simulink library "lib_electric_machine"  (Simulink 4.1.1)
undefined symbols (not defined in the file or in its folder): amb_tmp, cyc_mph, ess_module_num, ess_voc, fd_ratio, gb_num_init, gb_ratio, gc_cp, gc_inertia, gc_inpwr_map, gc_map_spd, gc_map_trq, gc_mass, gc_max_crrnt, gc_max_trq, gc_outpwr_map, gc_overtrq_factor, gc_sarea, gc_spd_scale, gc_th_calc, gc_trq_scale, gc_tstat, mc_cp, mc_eff_scale, mc_inertia, mc_init_tmp, mc_inpwr_map, mc_map_spd, mc_map_trq, mc_mass, mc_max_gen_trq, mc_max_trq, mc_overtrq_factor, mc_sarea, mc_spd_scale, mc_th_calc, mc_trq_scale, mc_tstat, tc_mc_to_fc_ratio, veh_mass, wh_radius
libraries: lib_electric_machine x4
(part 1 of 2)
settings Model: LastModifiedBy=ssprik
settings Model: ModifiedComment=|
  | abrooker -- Wed Aug 13 10:56:21 2003 -- Version 1.20
  | changed mc_eff_scale implementation into model
settings Model: ModifiedHistory=|
  | abrooker -- Tue Feb 04 10:35:40 2003 -- Version 1.19
  | added pwr goto for Altia
  | 
  | mokeefe -- Thu Apr 18 08:27:13 2002 -- Version 1.18
  | saving the model:
  | o "without the model browser open"
  | o with only top-level screen visible
  | o with "fit to view" enabled
  | o with "status bar" off and "toolbar" off
  | o with "prompt to update model history with each save" on

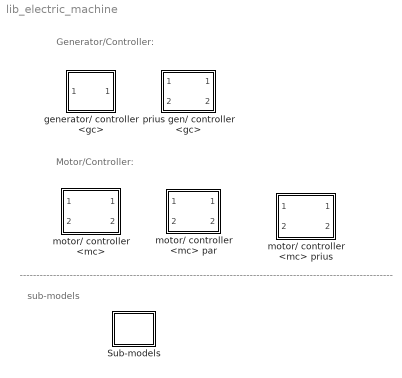
== system lib_electric_machine ==
  note: Generator/Controller:
  note: Motor/Controller:
  note: ----------------------------------------------------------------------------------------------------------------
  note: sub-models
  Sub-models : Subsystem
      settings: RTWFcnNameOpts=Auto  RTWFileNameOpts=Auto
  generator/ controller <gc> : Subsystem
      settings: RTWFcnNameOpts=Auto  RTWFileNameOpts=Auto
      mask Display: image(imread('bdi_mc.jpg'))
  motor/ controller <mc> : Subsystem
      settings: RTWFcnNameOpts=Auto  RTWFileNameOpts=Auto
      mask Display: image(imread('bdi_mc.jpg'))
  motor/ controller <mc> par : Subsystem
      settings: RTWFcnNameOpts=Auto  RTWFileNameOpts=Auto
      mask Display: image(imread('bdi_mc.jpg'))
  motor/ controller <mc> prius : Subsystem
      settings: RTWFcnNameOpts=Auto  RTWFileNameOpts=Auto
      mask Display: image(imread('bdi_mc.jpg'))
  prius gen/ controller <gc> : Subsystem
      settings: RTWFcnNameOpts=Auto  RTWFileNameOpts=Auto
      mask Display: image(imread('bdi_mc.jpg'))

== system lib_electric_machine/Sub-models ==
  motor inertia as a function of total vehicle inertia (generous approximation) : Subsystem  Orientation=up
      settings: RTWFcnNameOpts=Auto  RTWFileNameOpts=Auto
  veh mass calc : Subsystem
      settings: RTWFcnNameOpts=Auto  RTWFileNameOpts=Auto

== system lib_electric_machine/generator/ controller <gc> ==
  "torque and speed supplied to rotor (Nm), (rad/s)" : Inport  Port=1  LatchInput=off
  >=0 : Saturate  UpperLimit=inf  LowerLimit=0  LinearizeAsGain=on
  Block NOTES : Subsystem
      settings: RTWFcnNameOpts=Auto  RTWFileNameOpts=Auto
      mask Display: disp('Block\nNOTES')
  Demux : Demux  Outputs=2  BusSelectionMode=off
  Memory : Memory  X0=ess_module_num*mean(ess_voc(1,:))  InheritSampleTime=off
      settings: RTWStateStorageClass=Auto
  Sum : Sum  Inputs=+-  SaturateOnIntegerOverflow=on
  To Workspace9 : ToWorkspace  VariableName=gc_pwr_out_a  SampleTime=-1  SaveFormat=Array
      settings: Orientation=down
  effect of inertia (Nm) : Subsystem
      settings: RTWFcnNameOpts=Auto  RTWFileNameOpts=Auto
  enforce torque limit : Subsystem
      settings: RTWFcnNameOpts=Auto  RTWFileNameOpts=Auto
  enforce max speed : Saturate  UpperLimit=max(gc_map_spd)*gc_spd_scale  LowerLimit=0  LinearizeAsGain=on
  generator output power map (W) : Lookup2D  RowIndex=gc_map_spd*gc_spd_scale  ColumnIndex=gc_map_trq*gc_trq_scale  OutputValues=gc_outpwr_map*gc_spd_scale*gc_trq_scale
  help : Subsystem
      settings: OpenFcn=web(['file:\\\' which('generator_controller.htm')]);  RTWFcnNameOpts=Auto  RTWFileNameOpts=Auto
      mask Display: image(imread('doc_man.jpg'))
  limit request: controller current limit : Subsystem
      settings: RTWFcnNameOpts=Auto  RTWFileNameOpts=Auto
  generator output power (W) : Outport  Port=1  InitialOutput=0
  tag scope: gc_pwr_out_a=global, gc_spd_in_a=global, gc_trq_in_a=global
  wires:
  >=0/1 -> generator output power (W)/1, To Workspace9/1, [gc_pwr_out_a]
  limit request: controller current limit/1(out_1) -> >=0/1
  Demux/1 -> Sum/1, [gc_trq_in_a]
  [bus_voltage] -> Memory/1
  enforce max speed/1 -> generator output power map (W)/1, enforce torque limit/2(limited generator speed (rad/s))
  generator output power map (W)/1 -> limit request: controller current limit/1(computed output power (W))
  Sum/1 -> enforce torque limit/1(req'd generator input torque (Nm))
  enforce torque limit/1(limited generator input torque (Nm)) -> generator output power map (W)/2
  effect of inertia (Nm)/1(out_1) -> Sum/2
  Memory/1 -> limit request: controller current limit/2(bus voltage (V))
  "torque and speed supplied to rotor (Nm), (rad/s)"/1 -> Demux/1
  Demux/2 -> effect of inertia (Nm)/1(in_1), enforce max speed/1, [gc_spd_in_a]

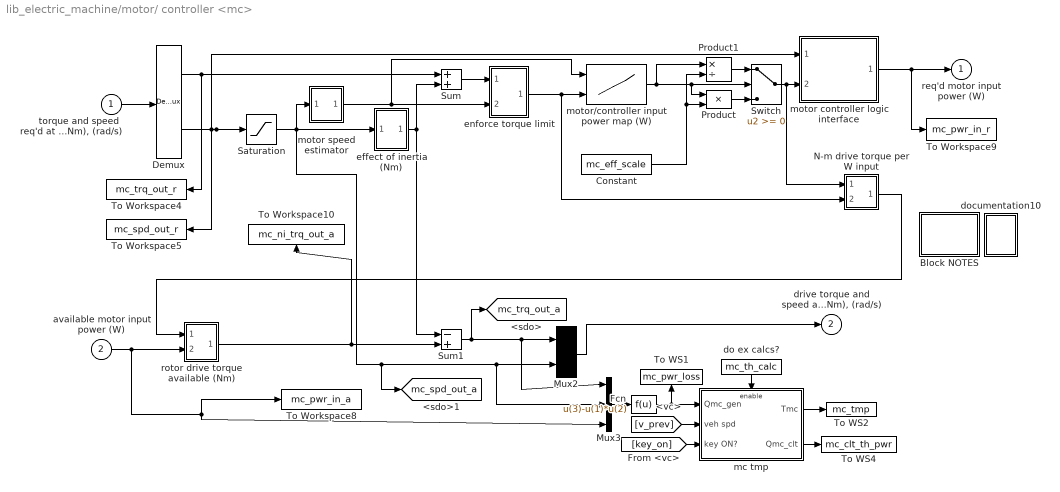
== system lib_electric_machine/motor/ controller <mc> ==
  "torque and speed  req'd at rotor (Nm), (rad/s)" : Inport  Port=1  LatchInput=off
  available motor input power (W) : Inport  Port=2  LatchInput=off
  Block NOTES : Subsystem
      settings: RTWFcnNameOpts=Auto  RTWFileNameOpts=Auto
      mask Display: disp('Block\nNOTES')
  Constant : Constant  Value=mc_eff_scale
  Demux : Demux  Outputs=2  BusSelectionMode=off
  Fcn : Fcn  Expr=u(3)-u(1)*u(2)
  Mux2 : Mux  Inputs=2
      settings: DisplayOption=none
  Mux3 : Mux  Inputs=3
      settings: DisplayOption=none
  N-m drive torque per W input : Subsystem
      settings: RTWFcnNameOpts=Auto  RTWFileNameOpts=Auto
  Product : Product  Inputs=2  Multiplication=Element-wise(.*)  SaturateOnIntegerOverflow=on
  Product1 : Product  Inputs=*/  Multiplication=Element-wise(.*)  SaturateOnIntegerOverflow=on
  Saturation : Saturate  UpperLimit=max(mc_map_spd)*mc_spd_scale  LowerLimit=0  LinearizeAsGain=on
  Sum : Sum  Inputs=++  SaturateOnIntegerOverflow=on
  Sum1 : Sum  Inputs=-+  SaturateOnIntegerOverflow=on
  Switch : Switch  Threshold=0
  To WS1 : ToWorkspace  VariableName=mc_pwr_loss  SampleTime=0  SaveFormat=Array
      settings: Orientation=up  MaxDataPoints=50000
  To WS2 : ToWorkspace  VariableName=mc_tmp  SampleTime=0  SaveFormat=Array
      settings: MaxDataPoints=50000
  To WS4 : ToWorkspace  VariableName=mc_clt_th_pwr  SampleTime=0  SaveFormat=Array
      settings: MaxDataPoints=50000
  To Workspace10 : ToWorkspace  VariableName=mc_ni_trq_out_a  SampleTime=-1  SaveFormat=Array
      settings: Orientation=up
  To Workspace4 : ToWorkspace  VariableName=mc_trq_out_r  SampleTime=-1  SaveFormat=Array
  To Workspace5 : ToWorkspace  VariableName=mc_spd_out_r  SampleTime=-1  SaveFormat=Array
  To Workspace8 : ToWorkspace  VariableName=mc_pwr_in_a  SampleTime=-1  SaveFormat=Array
  To Workspace9 : ToWorkspace  VariableName=mc_pwr_in_r  SampleTime=-1  SaveFormat=Array
  do ex calcs? : Constant  Orientation=down  Value=mc_th_calc
  documentation10 : Subsystem
      settings: OpenFcn=web(['file:\\\' which('motor_controller.htm')]);  RTWFcnNameOpts=Auto  RTWFileNameOpts=Auto
      mask Display: image(imread('doc_man.jpg'))
  effect of inertia (Nm) : Subsystem
      settings: RTWFcnNameOpts=Auto  RTWFileNameOpts=Auto
  enforce torque limit : Subsystem
      settings: RTWFcnNameOpts=Auto  RTWFileNameOpts=Auto
  mc tmp : Subsystem  TreatAsAtomicUnit=on
      settings: RTWFcnNameOpts=Auto  RTWFileNameOpts=Auto
  motor controller logic interface : Subsystem
      settings: RTWFcnNameOpts=Auto  RTWFileNameOpts=Auto
  motor speed estimator : Subsystem
      settings: RTWFcnNameOpts=Auto  RTWFileNameOpts=Auto
  motor/controller input power map (W) : Lookup2D  RowIndex=mc_map_spd*mc_spd_scale  ColumnIndex=mc_map_trq*mc_trq_scale  OutputValues=mc_inpwr_map*mc_spd_scale*mc_trq_scale
  rotor drive torque available (Nm) : Subsystem
      settings: RTWFcnNameOpts=Auto  RTWFileNameOpts=Auto
  req'd motor input power (W) : Outport  Port=1  InitialOutput=0
  "drive torque and speed avail. at rotor (Nm), (rad/s)" : Outport  Port=2  InitialOutput=0
  tag scope: mc_spd_out_a=global, mc_trq_out_a=global
  wires:
  "torque and speed  req'd at rotor (Nm), (rad/s)"/1 -> Demux/1
  Demux/1 -> To Workspace4/1, Sum/1
  available motor input power (W)/1 -> rotor drive torque available (Nm)/2(available input power (W)), To Workspace8/1, Mux3/3
  Demux/2 -> motor controller logic interface/1(w_mc_out_r), To Workspace5/1, Saturation/1
  [key_on] -> mc tmp/3(key ON?)
  [v_prev] -> mc tmp/2(veh spd)
  mc tmp/2(Qmc_clt) -> To WS4/1
  mc tmp/1(Tmc) -> To WS2/1
  do ex calcs?/1 -> mc tmp/Enable
  Fcn/1 -> mc tmp/1(Qmc_gen), To WS1/1
  Mux3/1 -> Fcn/1
  Mux2/1 -> "drive torque and speed avail. at rotor (Nm), (rad/s)"/1
  motor controller logic interface/1(P_mc_in_r) -> req'd motor input power (W)/1, To Workspace9/1
  enforce torque limit/1(limited motor torque (Nm)) -> N-m drive torque per W input/2(req'd rotor drive torque (Nm)), motor/controller input power map (W)/2
  effect of inertia (Nm)/1(out_1) -> Sum1/1, Sum/2
  Sum/1 -> enforce torque limit/1(req'd motor torque (Nm))
  Sum1/1 -> [mc_trq_out_a], Mux2/1, Mux3/1
  Saturation/1 -> motor speed estimator/1(mc_spd_out_a), effect of inertia (Nm)/1(mc_spd_out_a), [mc_spd_out_a], Mux2/2, Mux3/2
  motor speed estimator/1(Out1) -> enforce torque limit/2(limited motor speed (rad/s)), motor/controller input power map (W)/1
  N-m drive torque per W input/1(Nm per W) -> rotor drive torque available (Nm)/1(torque per unit input power (N-m/W))
  rotor drive torque available (Nm)/1(rotor drive torque available) -> To Workspace10/1, Sum1/2
  Switch/1 -> motor controller logic interface/2(P_mc_in_1lim), N-m drive torque per W input/1(req'd input power (W))
  Product1/1 -> Switch/1
  motor/controller input power map (W)/1 -> Product1/1, Switch/2, Product/1
  Constant/1 -> Product1/2, Product/2
  Product/1 -> Switch/3

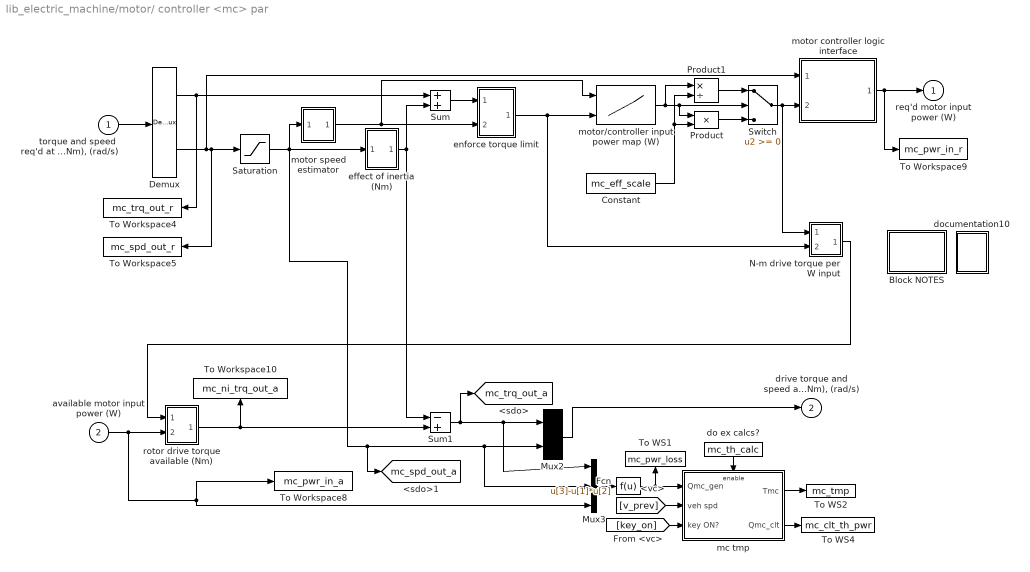
== system lib_electric_machine/motor/ controller <mc> par ==
  "torque and speed  req'd at rotor (Nm), (rad/s)" : Inport  Port=1  LatchInput=off
  available motor input power (W) : Inport  Port=2  LatchInput=off
  Block NOTES : Subsystem
      settings: RTWFcnNameOpts=Auto  RTWFileNameOpts=Auto
      mask Display: disp('Block\nNOTES')
  Constant : Constant  Value=mc_eff_scale
  Demux : Demux  Outputs=2  BusSelectionMode=off
  Fcn : Fcn  Expr=u[3]-u[1]*u[2]
  Mux2 : Mux  Inputs=2
      settings: DisplayOption=none
  Mux3 : Mux  Inputs=3
      settings: DisplayOption=none
  N-m drive torque per W input : Subsystem
      settings: RTWFcnNameOpts=Auto  RTWFileNameOpts=Auto
  Product : Product  Inputs=2  Multiplication=Element-wise(.*)  SaturateOnIntegerOverflow=on
  Product1 : Product  Inputs=*/  Multiplication=Element-wise(.*)  SaturateOnIntegerOverflow=on
  Saturation : Saturate  UpperLimit=max(mc_map_spd)*mc_spd_scale  LowerLimit=0  LinearizeAsGain=on
  Sum : Sum  Inputs=++  SaturateOnIntegerOverflow=on
  Sum1 : Sum  Inputs=-+  SaturateOnIntegerOverflow=on
  Switch : Switch  Threshold=0
  To WS1 : ToWorkspace  VariableName=mc_pwr_loss  SampleTime=0  SaveFormat=Array
      settings: Orientation=up  MaxDataPoints=50000
  To WS2 : ToWorkspace  VariableName=mc_tmp  SampleTime=0  SaveFormat=Array
      settings: MaxDataPoints=50000
  To WS4 : ToWorkspace  VariableName=mc_clt_th_pwr  SampleTime=0  SaveFormat=Array
      settings: MaxDataPoints=50000
  To Workspace10 : ToWorkspace  VariableName=mc_ni_trq_out_a  SampleTime=-1  SaveFormat=Array
      settings: Orientation=up
  To Workspace4 : ToWorkspace  VariableName=mc_trq_out_r  SampleTime=-1  SaveFormat=Array
  To Workspace5 : ToWorkspace  VariableName=mc_spd_out_r  SampleTime=-1  SaveFormat=Array
  To Workspace8 : ToWorkspace  VariableName=mc_pwr_in_a  SampleTime=-1  SaveFormat=Array
  To Workspace9 : ToWorkspace  VariableName=mc_pwr_in_r  SampleTime=-1  SaveFormat=Array
  do ex calcs? : Constant  Orientation=down  Value=mc_th_calc
  documentation10 : Subsystem
      settings: OpenFcn=web(['file:\\\' which('motor_controller.htm')]);  RTWFcnNameOpts=Auto  RTWFileNameOpts=Auto
      mask Display: image(imread('doc_man.jpg'))
  effect of inertia (Nm) : Subsystem
      settings: RTWFcnNameOpts=Auto  RTWFileNameOpts=Auto
  enforce torque limit : Subsystem
      settings: RTWFcnNameOpts=Auto  RTWFileNameOpts=Auto
  mc tmp : Subsystem  TreatAsAtomicUnit=on
      settings: RTWFcnNameOpts=Auto  RTWFileNameOpts=Auto
  motor controller logic interface : Subsystem
      settings: RTWFcnNameOpts=Auto  RTWFileNameOpts=Auto
  motor speed estimator : Subsystem
      settings: RTWFcnNameOpts=Auto  RTWFileNameOpts=Auto
  motor/controller input power map (W) : Lookup2D  RowIndex=mc_map_spd*mc_spd_scale  ColumnIndex=mc_map_trq*mc_trq_scale  OutputValues=mc_inpwr_map*mc_spd_scale*mc_trq_scale
  rotor drive torque available (Nm) : Subsystem
      settings: RTWFcnNameOpts=Auto  RTWFileNameOpts=Auto
  req'd motor input power (W) : Outport  Port=1  InitialOutput=0
  "drive torque and speed avail. at rotor (Nm), (rad/s)" : Outport  Port=2  InitialOutput=0
  tag scope: mc_spd_out_a=global, mc_trq_out_a=global
  wires:
  rotor drive torque available (Nm)/1(rotor drive torque available) -> To Workspace10/1, Sum1/2
  "torque and speed  req'd at rotor (Nm), (rad/s)"/1 -> Demux/1
  Demux/1 -> To Workspace4/1, Sum/1
  available motor input power (W)/1 -> rotor drive torque available (Nm)/2(available input power (W)), To Workspace8/1, Mux3/3
  Demux/2 -> motor controller logic interface/1(w_mc_out_r), To Workspace5/1, Saturation/1
  [key_on] -> mc tmp/3(key ON?)
  [v_prev] -> mc tmp/2(veh spd)
  mc tmp/2(Qmc_clt) -> To WS4/1
  mc tmp/1(Tmc) -> To WS2/1
  do ex calcs?/1 -> mc tmp/Enable
  Fcn/1 -> mc tmp/1(Qmc_gen), To WS1/1
  Mux3/1 -> Fcn/1
  Mux2/1 -> "drive torque and speed avail. at rotor (Nm), (rad/s)"/1
  motor controller logic interface/1(P_mc_in_r) -> req'd motor input power (W)/1, To Workspace9/1
  enforce torque limit/1(limited motor torque (Nm)) -> motor/controller input power map (W)/2, N-m drive torque per W input/2(req'd rotor drive torque (Nm))
  effect of inertia (Nm)/1(out_1) -> Sum1/1, Sum/2
  Sum/1 -> enforce torque limit/1(req'd motor torque (Nm))
  N-m drive torque per W input/1(Nm per W) -> rotor drive torque available (Nm)/1(torque per unit input power (N-m/W))
  Sum1/1 -> [mc_trq_out_a], Mux2/1, Mux3/1
  Saturation/1 -> [mc_spd_out_a], Mux2/2, Mux3/2, motor speed estimator/1(mc_spd_out_a), effect of inertia (Nm)/1(mc_spd_out_a)
  motor speed estimator/1(Out1) -> enforce torque limit/2(limited motor speed (rad/s)), motor/controller input power map (W)/1
  Constant/1 -> Product1/2, Product/2
  Switch/1 -> motor controller logic interface/2(P_mc_in_1lim), N-m drive torque per W input/1(req'd input power (W))
  Product1/1 -> Switch/1
  Product/1 -> Switch/3
  motor/controller input power map (W)/1 -> Product1/1, Switch/2, Product/1

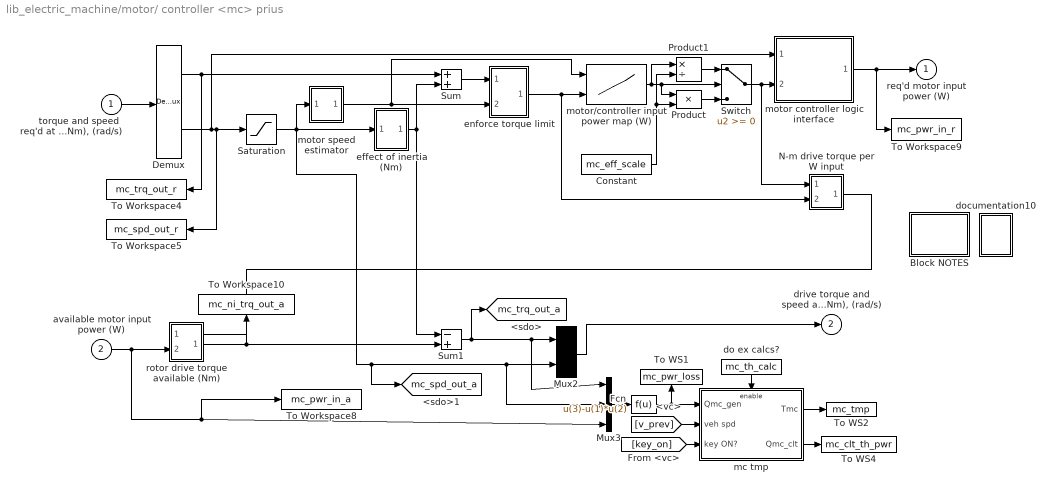
== system lib_electric_machine/motor/ controller <mc> prius ==
  "torque and speed  req'd at rotor (Nm), (rad/s)" : Inport  Port=1  LatchInput=off
  available motor input power (W) : Inport  Port=2  LatchInput=off
  Block NOTES : Subsystem
      settings: RTWFcnNameOpts=Auto  RTWFileNameOpts=Auto
      mask Display: disp('Block\nNOTES')
  Constant : Constant  Value=mc_eff_scale
  Demux : Demux  Outputs=2  BusSelectionMode=off
  Fcn : Fcn  Expr=u(3)-u(1)*u(2)
  Mux2 : Mux  Inputs=2
      settings: DisplayOption=none
  Mux3 : Mux  Inputs=3
      settings: DisplayOption=none
  N-m drive torque per W input : Subsystem
      settings: RTWFcnNameOpts=Auto  RTWFileNameOpts=Auto
  Product : Product  Inputs=2  Multiplication=Element-wise(.*)  SaturateOnIntegerOverflow=on
  Product1 : Product  Inputs=*/  Multiplication=Element-wise(.*)  SaturateOnIntegerOverflow=on
  Saturation : Saturate  UpperLimit=max(mc_map_spd)*mc_spd_scale  LowerLimit=0  LinearizeAsGain=on
  Sum : Sum  Inputs=++  SaturateOnIntegerOverflow=on
  Sum1 : Sum  Inputs=-+  SaturateOnIntegerOverflow=on
  Switch : Switch  Threshold=0
  To WS1 : ToWorkspace  VariableName=mc_pwr_loss  SampleTime=0  SaveFormat=Array
      settings: Orientation=up  MaxDataPoints=50000
  To WS2 : ToWorkspace  VariableName=mc_tmp  SampleTime=0  SaveFormat=Array
      settings: MaxDataPoints=50000
  To WS4 : ToWorkspace  VariableName=mc_clt_th_pwr  SampleTime=0  SaveFormat=Array
      settings: MaxDataPoints=50000
  To Workspace10 : ToWorkspace  VariableName=mc_ni_trq_out_a  SampleTime=-1  SaveFormat=Array
      settings: Orientation=up
  To Workspace4 : ToWorkspace  VariableName=mc_trq_out_r  SampleTime=-1  SaveFormat=Array
  To Workspace5 : ToWorkspace  VariableName=mc_spd_out_r  SampleTime=-1  SaveFormat=Array
  To Workspace8 : ToWorkspace  VariableName=mc_pwr_in_a  SampleTime=-1  SaveFormat=Array
  To Workspace9 : ToWorkspace  VariableName=mc_pwr_in_r  SampleTime=-1  SaveFormat=Array
  do ex calcs? : Constant  Orientation=down  Value=mc_th_calc
  documentation10 : Subsystem
      settings: OpenFcn=web(['file:\\\' which('motor_controller.htm')]);  RTWFcnNameOpts=Auto  RTWFileNameOpts=Auto
      mask Display: image(imread('doc_man.jpg'))
  effect of inertia (Nm) : Subsystem
      settings: RTWFcnNameOpts=Auto  RTWFileNameOpts=Auto
  enforce torque limit : Subsystem
      settings: RTWFcnNameOpts=Auto  RTWFileNameOpts=Auto
  mc tmp : Subsystem  TreatAsAtomicUnit=on
      settings: RTWFcnNameOpts=Auto  RTWFileNameOpts=Auto
  motor controller logic interface : Subsystem
      settings: RTWFcnNameOpts=Auto  RTWFileNameOpts=Auto
  motor speed estimator : Subsystem
      settings: RTWFcnNameOpts=Auto  RTWFileNameOpts=Auto
  motor/controller input power map (W) : Lookup2D  RowIndex=mc_map_spd*mc_spd_scale  ColumnIndex=mc_map_trq*mc_trq_scale  OutputValues=mc_inpwr_map*mc_spd_scale*mc_trq_scale
  rotor drive torque available (Nm) : Subsystem
      settings: RTWFcnNameOpts=Auto  RTWFileNameOpts=Auto
  req'd motor input power (W) : Outport  Port=1  InitialOutput=0
  "drive torque and speed avail. at rotor (Nm), (rad/s)" : Outport  Port=2  InitialOutput=0
  tag scope: mc_spd_out_a=global, mc_trq_out_a=global
  wires:
  rotor drive torque available (Nm)/1(rotor drive torque available) -> To Workspace10/1, Sum1/2
  "torque and speed  req'd at rotor (Nm), (rad/s)"/1 -> Demux/1
  Demux/1 -> To Workspace4/1, Sum/1
  available motor input power (W)/1 -> rotor drive torque available (Nm)/2(available input power (W)), To Workspace8/1, Mux3/3
  Demux/2 -> motor controller logic interface/1(w_mc_out_r), To Workspace5/1, Saturation/1
  [key_on] -> mc tmp/3(key ON?)
  [v_prev] -> mc tmp/2(veh spd)
  mc tmp/2(Qmc_clt) -> To WS4/1
  mc tmp/1(Tmc) -> To WS2/1
  do ex calcs?/1 -> mc tmp/Enable
  Fcn/1 -> mc tmp/1(Qmc_gen), To WS1/1
  Mux3/1 -> Fcn/1
  Mux2/1 -> "drive torque and speed avail. at rotor (Nm), (rad/s)"/1
  motor controller logic interface/1(P_mc_in_r) -> req'd motor input power (W)/1, To Workspace9/1
  enforce torque limit/1(limited motor torque (Nm)) -> N-m drive torque per W input/2(req'd rotor drive torque (Nm)), motor/controller input power map (W)/2
  effect of inertia (Nm)/1(out_1) -> Sum1/1, Sum/2
  Sum/1 -> enforce torque limit/1(req'd motor torque (Nm))
  N-m drive torque per W input/1(Nm per W) -> rotor drive torque available (Nm)/1(torque per unit input power (N-m/W))
  Sum1/1 -> [mc_trq_out_a], Mux2/1, Mux3/1
  Saturation/1 -> [mc_spd_out_a], Mux2/2, Mux3/2, motor speed estimator/1(mc_spd_out_a), effect of inertia (Nm)/1(mc_spd_out_a)
  motor speed estimator/1(Out1) -> enforce torque limit/2(limited motor speed (rad/s)), motor/controller input power map (W)/1
  Product/1 -> Switch/3
  motor/controller input power map (W)/1 -> Product1/1, Switch/2, Product/1
  Switch/1 -> motor controller logic interface/2(P_mc_in_1lim), N-m drive torque per W input/1(req'd input power (W))
  Product1/1 -> Switch/1
  Constant/1 -> Product1/2, Product/2

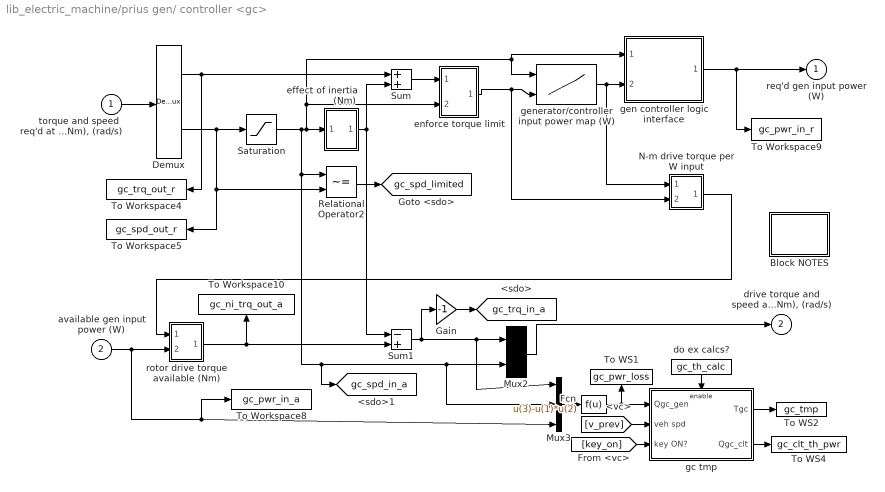
== system lib_electric_machine/prius gen/ controller <gc> ==
  "torque and speed  req'd at rotor (Nm), (rad/s)" : Inport  Port=1  LatchInput=off
  available gen input power (W) : Inport  Port=2  LatchInput=off
  Block NOTES : Subsystem
      settings: RTWFcnNameOpts=Auto  RTWFileNameOpts=Auto
      mask Display: disp('Block\nNOTES')
  Demux : Demux  Outputs=2  BusSelectionMode=off
  Fcn : Fcn  Expr=u(3)-u(1)*u(2)
  Gain : Gain  Gain=-1  Multiplication=Element-wise(K.*u)  SaturateOnIntegerOverflow=on
  Mux2 : Mux  Inputs=2
      settings: DisplayOption=none
  Mux3 : Mux  Inputs=3
      settings: DisplayOption=none
  N-m drive torque per W input : Subsystem
      settings: RTWFcnNameOpts=Auto  RTWFileNameOpts=Auto
  Relational Operator2 : RelationalOperator  Operator=~=
  Saturation : Saturate  UpperLimit=max(gc_map_spd)*gc_spd_scale  LowerLimit=-max(gc_map_spd)*gc_spd_scale  LinearizeAsGain=on
  Sum : Sum  Inputs=++  SaturateOnIntegerOverflow=on
  Sum1 : Sum  Inputs=-+  SaturateOnIntegerOverflow=on
  To WS1 : ToWorkspace  VariableName=gc_pwr_loss  SampleTime=0  SaveFormat=Array
      settings: Orientation=up
  To WS2 : ToWorkspace  VariableName=gc_tmp  SampleTime=0  SaveFormat=Array
  To WS4 : ToWorkspace  VariableName=gc_clt_th_pwr  SampleTime=0  SaveFormat=Array
  To Workspace10 : ToWorkspace  VariableName=gc_ni_trq_out_a  SampleTime=-1  SaveFormat=Array
      settings: Orientation=up
  To Workspace4 : ToWorkspace  VariableName=gc_trq_out_r  SampleTime=-1  SaveFormat=Array
  To Workspace5 : ToWorkspace  VariableName=gc_spd_out_r  SampleTime=-1  SaveFormat=Array
  To Workspace8 : ToWorkspace  VariableName=gc_pwr_in_a  SampleTime=-1  SaveFormat=Array
  To Workspace9 : ToWorkspace  VariableName=gc_pwr_in_r  SampleTime=-1  SaveFormat=Array
  do ex calcs? : Constant  Orientation=down  Value=gc_th_calc
  effect of inertia (Nm) : Subsystem
      settings: RTWFcnNameOpts=Auto  RTWFileNameOpts=Auto
  enforce torque limit : Subsystem
      settings: RTWFcnNameOpts=Auto  RTWFileNameOpts=Auto
  gc tmp : Subsystem  TreatAsAtomicUnit=on
      settings: RTWFcnNameOpts=Auto  RTWFileNameOpts=Auto
  gen controller logic interface : Subsystem
      settings: RTWFcnNameOpts=Auto  RTWFileNameOpts=Auto
  generator/controller input power map (W) : Lookup2D  RowIndex=gc_map_spd*gc_spd_scale  ColumnIndex=gc_map_trq*gc_trq_scale  OutputValues=gc_inpwr_map*gc_spd_scale*gc_trq_scale
  rotor drive torque available (Nm) : Subsystem
      settings: RTWFcnNameOpts=Auto  RTWFileNameOpts=Auto
  req'd gen input power (W) : Outport  Port=1  InitialOutput=0
  "drive torque and speed avail. at rotor (Nm), (rad/s)" : Outport  Port=2  InitialOutput=0
  tag scope: gc_spd_in_a=global, gc_spd_limited=global, gc_trq_in_a=global
  wires:
  [key_on] -> gc tmp/3(key ON?)
  [v_prev] -> gc tmp/2(veh spd)
  gc tmp/2(Qgc_clt) -> To WS4/1
  gc tmp/1(Tgc) -> To WS2/1
  do ex calcs?/1 -> gc tmp/Enable
  Fcn/1 -> gc tmp/1(Qgc_gen), To WS1/1
  Mux3/1 -> Fcn/1
  Mux2/1 -> "drive torque and speed avail. at rotor (Nm), (rad/s)"/1
  generator/controller input power map (W)/1 -> N-m drive torque per W input/1(req'd input power (W)), gen controller logic interface/2(P_gc_in_1lim)
  rotor drive torque available (Nm)/1(rotor drive torque available) -> To Workspace10/1, Sum1/2
  "torque and speed  req'd at rotor (Nm), (rad/s)"/1 -> Demux/1
  enforce torque limit/1(limited generator torque (Nm)) -> N-m drive torque per W input/2(req'd rotor drive torque (Nm)), generator/controller input power map (W)/2
  effect of inertia (Nm)/1(out_1) -> Sum1/1, Sum/2
  Sum/1 -> enforce torque limit/1(req'd gen torque (Nm))
  Saturation/1 -> effect of inertia (Nm)/1(in_1), gen controller logic interface/1(w_gc_out_r), generator/controller input power map (W)/1, enforce torque limit/2(limited gen speed (rad/s)), Relational Operator2/1, [gc_spd_in_a], Mux2/2, Mux3/2
  Relational Operator2/1 -> [gc_spd_limited]
  Demux/2 -> Saturation/1, Relational Operator2/2, To Workspace5/1
  N-m drive torque per W input/1(Nm per W) -> rotor drive torque available (Nm)/1(torque per unit input power (N-m/W))
  Demux/1 -> Sum/1, To Workspace4/1
  Sum1/1 -> Gain/1, Mux2/1, Mux3/1
  available gen input power (W)/1 -> rotor drive torque available (Nm)/2(available input power (W)), To Workspace8/1, Mux3/3
  gen controller logic interface/1(P_gc_in_r) -> To Workspace9/1, req'd gen input power (W)/1
  Gain/1 -> [gc_trq_in_a]

== system lib_electric_machine/Sub-models/motor inertia as a function of total vehicle inertia (generous approximation) ==
  gear ratio : Inport  Orientation=down  Port=1  LatchInput=off
  Product : Product  Orientation=down  Inputs=*/  Multiplication=Element-wise(.*)  SaturateOnIntegerOverflow=on
  Sum : Sum  Orientation=down  Inputs=++|  SaturateOnIntegerOverflow=on
  engine inertia as a fraction of total vehicle inertia  (generous approximation)--denomenator : Fcn  Orientation=down  Expr=mc_inertia*u^2
  engine inertia as a fraction of total vehicle inertia  (generous approximation)--numerator : Fcn  Orientation=down  Expr=mc_inertia*u^2
  veh mass calc : lib_electric_machine/Sub-models/veh mass calc
  Out1 : Outport  Orientation=down  Port=1
  wires:
  engine inertia as a fraction of total vehicle inertia  (generous approximation)--numerator/1 -> Product/1
  Product/1 -> Out1/1
  gear ratio/1 -> engine inertia as a fraction of total vehicle inertia  (generous approximation)--numerator/1, engine inertia as a fraction of total vehicle inertia  (generous approximation)--denomenator/1
  veh mass calc/1 -> Sum/1
  engine inertia as a fraction of total vehicle inertia  (generous approximation)--denomenator/1 -> Sum/2
  Sum/1 -> Product/2

== system lib_electric_machine/Sub-models/veh mass calc ==
  Constant : Constant  Value=veh_mass
  Sum : Sum  Inputs=|++  SaturateOnIntegerOverflow=on
  Out1 : Outport  Port=1
  wires:
  [veh_cargo_mass] -> Sum/1
  Constant/1 -> Sum/2
  Sum/1 -> Out1/1

== system lib_electric_machine/generator/ controller <gc>/Block NOTES ==
  note: This generator/controller model includes loss data, rotational inertia, and performance limits.
      | This is the only entirely forward-facing block in ADVISOR, computing the output power from the
      | input torque and speed.  The generator map used in the lookup table block is VERY similar to
      | the input power motor map, with the main difference being that the torque and power sign
      | conventions are opposite: here torque input to the machine and power output by the machine
      | are positive.

== system lib_electric_machine/generator/ controller <gc>/effect of inertia (Nm) ==
  in_1 : Inport  Port=1  LatchInput=off
  Gain : Gain  Gain=gc_inertia  Multiplication=Element-wise(K.*u)  SaturateOnIntegerOverflow=on
  alpha : Derivative
  out_1 : Outport  Port=1  InitialOutput=0
  wires:
  Gain/1 -> out_1/1
  alpha/1 -> Gain/1
  in_1/1 -> alpha/1

== system lib_electric_machine/generator/ controller <gc>/enforce torque limit ==
  req'd generator input torque (Nm) : Inport  Port=1  LatchInput=off
  limited generator speed (rad/s) : Inport  Port=2  LatchInput=off
  Block NOTES : Subsystem
      settings: RTWFcnNameOpts=Auto  RTWFileNameOpts=Auto
      mask Display: disp('Block\nNOTES')
  MinMax : MinMax  Function=min  Inputs=2
  max torque : Lookup  InputValues=gc_map_spd*gc_spd_scale  OutputValues=gc_max_trq*gc_overtrq_factor*gc_trq_scale
  limited generator input torque (Nm) : Outport  Port=1
  wires:
  limited generator speed (rad/s)/1 -> max torque/1
  MinMax/1 -> limited generator input torque (Nm)/1
  max torque/1 -> MinMax/2
  req'd generator input torque (Nm)/1 -> MinMax/1

== system lib_electric_machine/generator/ controller <gc>/help ==

== system lib_electric_machine/generator/ controller <gc>/limit request: controller current limit ==
  computed output power (W) : Inport  Port=1  LatchInput=off
  bus voltage (V) : Inport  Port=2  LatchInput=off
  Block NOTES : Subsystem
      settings: RTWFcnNameOpts=Auto  RTWFileNameOpts=Auto
      mask Display: disp('Block\nNOTES')
  Constant : Constant  Value=gc_max_crrnt
  MinMax : MinMax  Function=min  Inputs=2
  Product1 : Product  Inputs=2  Multiplication=Element-wise(.*)  SaturateOnIntegerOverflow=on
  out_1 : Outport  Port=1  InitialOutput=0
  wires:
  computed output power (W)/1 -> MinMax/1
  Product1/1 -> MinMax/2
  Constant/1 -> Product1/1
  bus voltage (V)/1 -> Product1/2
  MinMax/1 -> out_1/1

== system lib_electric_machine/motor/ controller <mc>/Block NOTES ==
  note: This motor/controller model includes loss data, rotational inertia, and performance limits.
  note: Available torque is computed from available power by assuming that the ratio of rotor torque to input
      | (electric) power is the same for the actual/achievable situation as was computed for the request.  This
      | is mathematically equivalent to assuming that the motor/controller efficiency.  Rotor speed for the
      | actual/achievable calculations is as computed in the 'request' branch.

== system lib_electric_machine/motor/ controller <mc>/N-m drive torque per W input ==
  req'd input power (W) : Inport  Port=1  LatchInput=off
  req'd rotor drive torque (Nm) : Inport  Port=2  LatchInput=off
  Block NOTES : Subsystem
      settings: RTWFcnNameOpts=Auto  RTWFileNameOpts=Auto
      mask Display: disp('Block\nNOTES')
  Constant : Constant  Value=eps
  Constant1 : Constant  Value=0
  Constant2 : Constant  Value=inf
  Product : Product  Inputs=/*  Multiplication=Element-wise(.*)  SaturateOnIntegerOverflow=on
  Relational Operator : RelationalOperator  Operator=~=
  Sum : Sum  Inputs=++  SaturateOnIntegerOverflow=on
  Switch : Switch  Threshold=eps
  Nm per W : Outport  Port=1  InitialOutput=0
  wires:
  Constant/1 -> Sum/1
  req'd rotor drive torque (Nm)/1 -> Product/2
  Product/1 -> Switch/1
  Relational Operator/1 -> Switch/2
  Switch/1 -> Nm per W/1
  Sum/1 -> Product/1
  req'd input power (W)/1 -> Sum/2, Relational Operator/1
  Constant1/1 -> Relational Operator/2
  Constant2/1 -> Switch/3

== system lib_electric_machine/motor/ controller <mc>/documentation10 ==

== system lib_electric_machine/motor/ controller <mc>/effect of inertia (Nm) ==
  mc_spd_out_a : Inport  Port=1  LatchInput=off
  Block NOTES : Subsystem
      settings: RTWFcnNameOpts=Auto  RTWFileNameOpts=Auto
      mask Display: disp('Block\nNOTES')
  Constant : Constant  Value=eps
  Constant1 : Constant  Value=max(mc_max_trq)*mc_trq_scale*mc_overtrq_factor
  Constant2 : Constant  Orientation=left  Value=gb_ratio(1)*fd_ratio/wh_radius
  Gain : Gain  Gain=mc_inertia  Multiplication=Element-wise(K.*u)  SaturateOnIntegerOverflow=on
  Memory : Memory  X0=0  InheritSampleTime=off
      settings: RTWStateStorageClass=Auto
  MinMax : MinMax  Function=min  Inputs=2
  Product : Product  Inputs=2  Multiplication=Element-wise(.*)  SaturateOnIntegerOverflow=on
  Sum : Sum  Inputs=++  SaturateOnIntegerOverflow=on
  Switch : Switch  Threshold=eps
  alpha : Derivative
  motor inertia as a fraction of total vehicle inertia (generous approximation) : lib_electric_machine/Sub-models/motor inertia as a function of total vehicle inertia (generous approximation)  Orientation=up
  overall gear ratio / wh_radius : Product  Inputs=*/  Multiplication=Element-wise(.*)  SaturateOnIntegerOverflow=on
  out_1 : Outport  Port=1  InitialOutput=0
  wires:
  alpha/1 -> Gain/1
  mc_spd_out_a/1 -> alpha/1, overall gear ratio / wh_radius/1
  MinMax/1 -> out_1/1
  Gain/1 -> MinMax/1
  Product/1 -> MinMax/2
  overall gear ratio / wh_radius/1 -> Memory/1
  Constant1/1 -> Product/1
  Memory/1 -> motor inertia as a fraction of total vehicle inertia (generous approximation)/1
  motor inertia as a fraction of total vehicle inertia (generous approximation)/1 -> Product/2
  Constant/1 -> Sum/2
  Sum/1 -> Switch/1
  [veh_spd_a_rec] -> Sum/1, Switch/2
  Constant2/1 -> Switch/3
  Switch/1 -> overall gear ratio / wh_radius/2

== system lib_electric_machine/motor/ controller <mc>/enforce torque limit ==
  req'd motor torque (Nm) : Inport  Port=1  LatchInput=off
  limited motor speed (rad/s) : Inport  Port=2  LatchInput=off
  Block NOTES : Subsystem
      settings: RTWFcnNameOpts=Auto  RTWFileNameOpts=Auto
      mask Display: disp('Block\nNOTES')
  MinMax : MinMax  Function=min  Inputs=2
  MinMax1 : MinMax  Function=max  Inputs=2
  Relational Operator2 : RelationalOperator  Operator=~=
  Switch : Switch  Threshold=0
  To WS2 : ToWorkspace  VariableName=mc_max_trq_vec  SampleTime=0  SaveFormat=Array
      settings: MaxDataPoints=50000
  max gen torque : Lookup  InputValues=mc_map_spd*mc_spd_scale  OutputValues=mc_max_gen_trq*mc_overtrq_factor*mc_trq_scale
  max torque : Lookup  InputValues=mc_map_spd*mc_spd_scale  OutputValues=mc_max_trq*mc_overtrq_factor*mc_trq_scale
  limited motor torque (Nm) : Outport  Port=1
  tag scope: mc_trq_limited=global
  wires:
  max torque/1 -> To WS2/1, MinMax/2
  req'd motor torque (Nm)/1 -> Relational Operator2/1, Switch/2, MinMax1/1, MinMax/1
  Switch/1 -> Relational Operator2/2, limited motor torque (Nm)/1
  MinMax1/1 -> Switch/3
  MinMax/1 -> Switch/1
  Relational Operator2/1 -> [mc_trq_limited]
  limited motor speed (rad/s)/1 -> max torque/1, max gen torque/1
  max gen torque/1 -> MinMax1/2

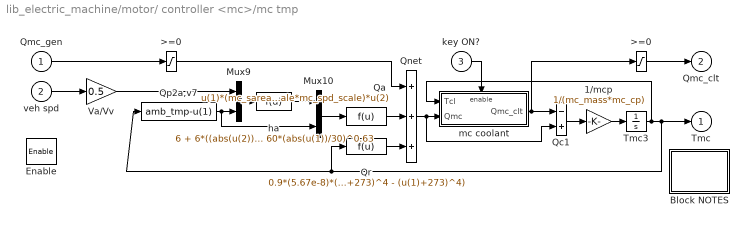
== system lib_electric_machine/motor/ controller <mc>/mc tmp ==
  Qmc_gen : Inport  Port=1  LatchInput=off
  veh spd : Inport  Port=2  LatchInput=off
  key ON? : Inport  Port=3  LatchInput=off
  Enable : EnablePort  StatesWhenEnabling=reset
  1/mcp : Gain  Gain=1/(mc_mass*mc_cp)  Multiplication=Element-wise(K.*u)  SaturateOnIntegerOverflow=on
  >=0 : Saturate  UpperLimit=Inf  LowerLimit=0  LinearizeAsGain=on
  ">=0 " : Saturate  UpperLimit=Inf  LowerLimit=0  LinearizeAsGain=on
  Block NOTES : Subsystem
      settings: RTWFcnNameOpts=Auto  RTWFileNameOpts=Auto
      mask Display: disp('Block\nNOTES')
  Mux10 : Mux  Inputs=2
      settings: DisplayOption=none
  Mux9 : Mux  Inputs=2
      settings: DisplayOption=none
  Qa : Fcn  Expr=u(1)*(mc_sarea*mc_trq_scale*mc_spd_scale)*u(2)
  Qc1 : Sum  Inputs=-+  SaturateOnIntegerOverflow=on
  Qnet : Sum  Inputs=+++  SaturateOnIntegerOverflow=on
  Qp2a,v7 : Fcn  Expr=amb_tmp-u(1)
  Qr : Fcn  Expr=0.9*(5.67e-8)*(mc_sarea*mc_trq_scale*mc_spd_scale)*((amb_tmp+273)^4 - (u(1)+273)^4)
  Tmc3 : Integrator  ExternalReset=none  InitialConditionSource=internal  InitialCondition=mc_init_tmp  LimitOutput=off  UpperSaturationLimit=inf  LowerSaturationLimit=-inf  ShowSaturationPort=off  ShowStatePort=off  AbsoluteTolerance=auto
  Va/Vv : Gain  Gain=0.5  Multiplication=Element-wise(K.*u)  SaturateOnIntegerOverflow=on
  ha : Fcn  Expr=6 + 6*((abs(u(2))/1000))^0.25 + 60*(abs(u(1))/30)^0.63
  mc coolant : Subsystem  TreatAsAtomicUnit=on
      settings: RTWFcnNameOpts=Auto  RTWFileNameOpts=Auto
  Tmc : Outport  Port=1  InitialOutput=0
  Qmc_clt : Outport  Port=2  OutputWhenDisabled=reset  InitialOutput=0
  wires:
  Mux10/1 -> Qa/1
  Mux9/1 -> ha/1
  Va/Vv/1 -> Mux9/1
  ha/1 -> Mux10/1
  Qp2a,v7/1 -> Mux9/2, Mux10/2
  Qr/1 -> Qnet/3
  Qmc_gen/1 -> ">=0 "/1
  ">=0 "/1 -> Qnet/1
  Qa/1 -> Qnet/2
  veh spd/1 -> Va/Vv/1
  key ON?/1 -> mc coolant/Enable
  >=0/1 -> Qmc_clt/1
  mc coolant/1(Qmc_clt) -> >=0/1, Qc1/1
  Tmc3/1 -> mc coolant/1(Tcl), Tmc/1, Qr/1, Qp2a,v7/1
  1/mcp/1 -> Tmc3/1
  Qc1/1 -> 1/mcp/1
  Qnet/1 -> mc coolant/2("Qmc "), Qc1/2

== system lib_electric_machine/motor/ controller <mc>/motor controller logic interface ==
  w_mc_out_r : Inport  Port=1  LatchInput=off
  P_mc_in_1lim : Inport  Port=2  LatchInput=off
  P_mc_in_r : Outport  Port=1  InitialOutput=0
  tag scope: P_mc_in_1lim=global, w_mc_out_r=global
  wires:
  P_mc_in_1lim/1 -> [P_mc_in_1lim]
  w_mc_out_r/1 -> [w_mc_out_r]
  [P_mc_in_r] -> P_mc_in_r/1

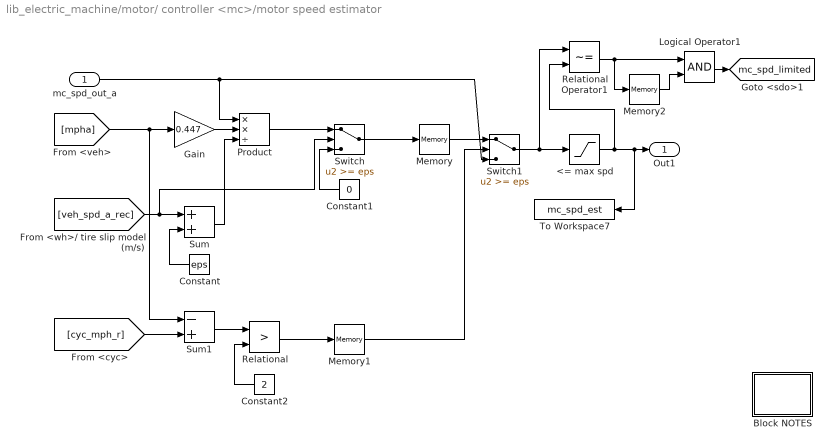
== system lib_electric_machine/motor/ controller <mc>/motor speed estimator ==
  mc_spd_out_a : Inport  Port=1  LatchInput=off
  <= max spd : Saturate  UpperLimit=max(mc_map_spd)*mc_spd_scale  LowerLimit=-inf  LinearizeAsGain=on
  Block NOTES : Subsystem
      settings: RTWFcnNameOpts=Auto  RTWFileNameOpts=Auto
      mask Display: disp('Block\nNOTES')
  Constant : Constant  Orientation=left  Value=eps
  Constant1 : Constant  Orientation=left  Value=0
  Constant2 : Constant  Orientation=left  Value=2
  Gain : Gain  Gain=0.447  Multiplication=Element-wise(K.*u)  SaturateOnIntegerOverflow=on
  Logical Operator1 : Logic  Operator=AND  Inputs=2
  Memory : Memory  X0=cyc_mph(1,2)*0.447/wh_radius*fd_ratio*gb_ratio(gb_num_init)  InheritSampleTime=off
      settings: RTWStateStorageClass=Auto
  Memory1 : Memory  X0=1  InheritSampleTime=off
      settings: RTWStateStorageClass=Auto
  Memory2 : Memory  X0=0  InheritSampleTime=off
      settings: RTWStateStorageClass=Auto
  Product : Product  Inputs=**/  Multiplication=Element-wise(.*)  SaturateOnIntegerOverflow=on
  Relational : RelationalOperator  Operator=>
  Relational Operator1 : RelationalOperator  Operator=~=
  Sum : Sum  Inputs=++  SaturateOnIntegerOverflow=on
  Sum1 : Sum  Inputs=-+  SaturateOnIntegerOverflow=on
  Switch : Switch  Threshold=eps
  Switch1 : Switch  Threshold=eps
  To Workspace7 : ToWorkspace  VariableName=mc_spd_est  SampleTime=-1  SaveFormat=Array
  Out1 : Outport  Port=1
  tag scope: mc_spd_limited=global
  wires:
  <= max spd/1 -> Relational Operator1/2, To Workspace7/1, Out1/1
  Switch1/1 -> Relational Operator1/1, <= max spd/1
  Relational Operator1/1 -> Memory2/1, Logical Operator1/1
  Logical Operator1/1 -> [mc_spd_limited]
  Memory2/1 -> Logical Operator1/2
  mc_spd_out_a/1 -> Switch1/3, Product/1
  Product/1 -> Switch/1
  Sum/1 -> Product/3
  Gain/1 -> Product/2
  [veh_spd_a_rec] -> Sum/1, Switch/2
  Constant1/1 -> Switch/3
  Memory/1 -> Switch1/1
  Constant/1 -> Sum/2
  [cyc_mph_r] -> Sum1/2
  [mpha] -> Gain/1, Sum1/1
  Constant2/1 -> Relational/2
  Sum1/1 -> Relational/1
  Relational/1 -> Memory1/1
  Memory1/1 -> Switch1/2
  Switch/1 -> Memory/1

== system lib_electric_machine/motor/ controller <mc>/rotor drive torque available (Nm) ==
  torque per unit input power (N-m/W) : Inport  Port=1  LatchInput=off
  available input power (W) : Inport  Port=2  LatchInput=off
  Block NOTES : Subsystem
      settings: RTWFcnNameOpts=Auto  RTWFileNameOpts=Auto
      mask Display: disp('Block\nNOTES')
  Constant2 : Constant  Value=inf
  Constant3 : Constant  Value=0
  Product : Product  Inputs=2  Multiplication=Element-wise(.*)  SaturateOnIntegerOverflow=on
  Relational Operator : RelationalOperator  Operator=~=
  Switch : Switch  Threshold=eps
  rotor drive torque available : Outport  Port=1  InitialOutput=0
  wires:
  Constant3/1 -> Switch/3
  Constant2/1 -> Relational Operator/2
  available input power (W)/1 -> Product/2
  Product/1 -> Switch/1
  Relational Operator/1 -> Switch/2
  Switch/1 -> rotor drive torque available/1
  torque per unit input power (N-m/W)/1 -> Product/1, Relational Operator/1

== system lib_electric_machine/motor/ controller <mc> par/Block NOTES ==
  note: This motor/controller model includes loss data, rotational inertia, and performance limits.
  note: Available torque is computed from available power by assuming that the ratio of rotor torque to input
      | (electric) power is the same for the actual/achievable situation as was computed for the request.  This
      | is mathematically equivalent to assuming that the motor/controller efficiency.  Rotor speed for the
      | actual/achievable calculations is as computed in the 'request' branch.

== system lib_electric_machine/motor/ controller <mc> par/N-m drive torque per W input ==
  req'd input power (W) : Inport  Port=1  LatchInput=off
  req'd rotor drive torque (Nm) : Inport  Port=2  LatchInput=off
  Block NOTES : Subsystem
      settings: RTWFcnNameOpts=Auto  RTWFileNameOpts=Auto
      mask Display: disp('Block\nNOTES')
  Constant : Constant  Value=eps
  Constant1 : Constant  Value=0
  Constant2 : Constant  Value=inf
  Product : Product  Inputs=/*  Multiplication=Element-wise(.*)  SaturateOnIntegerOverflow=on
  Relational Operator : RelationalOperator  Operator=~=
  Sum : Sum  Inputs=++  SaturateOnIntegerOverflow=on
  Switch : Switch  Threshold=eps
  Nm per W : Outport  Port=1  InitialOutput=0
  wires:
  Constant/1 -> Sum/1
  req'd rotor drive torque (Nm)/1 -> Product/2
  Product/1 -> Switch/1
  Relational Operator/1 -> Switch/2
  Switch/1 -> Nm per W/1
  Sum/1 -> Product/1
  req'd input power (W)/1 -> Sum/2, Relational Operator/1
  Constant1/1 -> Relational Operator/2
  Constant2/1 -> Switch/3

== system lib_electric_machine/motor/ controller <mc> par/documentation10 ==

== system lib_electric_machine/motor/ controller <mc> par/effect of inertia (Nm) ==
  mc_spd_out_a : Inport  Port=1  LatchInput=off
  Block NOTES : Subsystem
      settings: RTWFcnNameOpts=Auto  RTWFileNameOpts=Auto
      mask Display: disp('Block\nNOTES')
  Constant : Constant  Value=eps
  Constant1 : Constant  Value=max(mc_max_trq)*mc_trq_scale*mc_overtrq_factor
  Constant2 : Constant  Orientation=left  Value=gb_ratio(1)*fd_ratio/wh_radius
  Gain : Gain  Gain=mc_inertia  Multiplication=Element-wise(K.*u)  SaturateOnIntegerOverflow=on
  Memory : Memory  X0=0  InheritSampleTime=off
      settings: RTWStateStorageClass=Auto
  MinMax : MinMax  Function=min  Inputs=2
  Product : Product  Inputs=2  Multiplication=Element-wise(.*)  SaturateOnIntegerOverflow=on
  Sum : Sum  Inputs=++  SaturateOnIntegerOverflow=on
  Switch : Switch  Threshold=eps
  alpha : Derivative
  motor inertia as a function of total vehicle inertia (generous approximation) : lib_electric_machine/Sub-models/motor inertia as a function of total vehicle inertia (generous approximation)  Orientation=up
  overall gear ratio / wh_radius : Product  Inputs=*/  Multiplication=Element-wise(.*)  SaturateOnIntegerOverflow=on
  out_1 : Outport  Port=1  InitialOutput=0
  wires:
  alpha/1 -> Gain/1
  mc_spd_out_a/1 -> alpha/1, overall gear ratio / wh_radius/1
  MinMax/1 -> out_1/1
  Gain/1 -> MinMax/1
  Product/1 -> MinMax/2
  overall gear ratio / wh_radius/1 -> Memory/1
  Constant1/1 -> Product/1
  Memory/1 -> motor inertia as a function of total vehicle inertia (generous approximation)/1
  motor inertia as a function of total vehicle inertia (generous approximation)/1 -> Product/2
  Constant/1 -> Sum/2
  Sum/1 -> Switch/1
  [veh_spd_a_rec] -> Sum/1, Switch/2
  Constant2/1 -> Switch/3
  Switch/1 -> overall gear ratio / wh_radius/2

== system lib_electric_machine/motor/ controller <mc> par/enforce torque limit ==
  req'd motor torque (Nm) : Inport  Port=1  LatchInput=off
  limited motor speed (rad/s) : Inport  Port=2  LatchInput=off
  Block NOTES : Subsystem
      settings: RTWFcnNameOpts=Auto  RTWFileNameOpts=Auto
      mask Display: disp('Block\nNOTES')
  MinMax : MinMax  Function=min  Inputs=2
  MinMax1 : MinMax  Function=max  Inputs=2
  Relational Operator2 : RelationalOperator  Operator=~=
  Switch : Switch  Threshold=0
  To WS2 : ToWorkspace  VariableName=mc_max_trq_vec  SampleTime=0  SaveFormat=Array
      settings: MaxDataPoints=50000
  max gen torque : Lookup  InputValues=mc_map_spd*mc_spd_scale  OutputValues=mc_max_gen_trq*mc_overtrq_factor*mc_trq_scale
  max torque : Lookup  InputValues=mc_map_spd*mc_spd_scale  OutputValues=mc_max_trq*mc_overtrq_factor*mc_trq_scale
  limited motor torque (Nm) : Outport  Port=1
  tag scope: mc_trq_limited=global
  wires:
  max torque/1 -> To WS2/1, MinMax/2
  req'd motor torque (Nm)/1 -> Relational Operator2/1, Switch/2, MinMax1/1, MinMax/1
  Switch/1 -> Relational Operator2/2, limited motor torque (Nm)/1
  MinMax1/1 -> Switch/3
  MinMax/1 -> Switch/1
  Relational Operator2/1 -> [mc_trq_limited]
  limited motor speed (rad/s)/1 -> max torque/1, max gen torque/1
  max gen torque/1 -> MinMax1/2

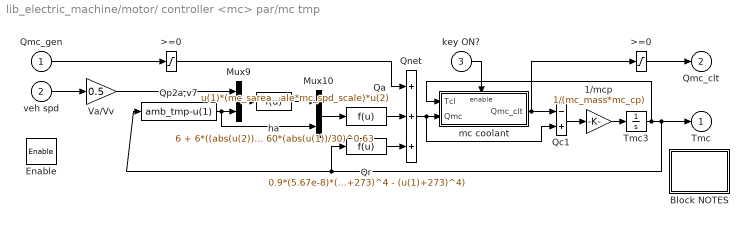
== system lib_electric_machine/motor/ controller <mc> par/mc tmp ==
  Qmc_gen : Inport  Port=1  LatchInput=off
  veh spd : Inport  Port=2  LatchInput=off
  key ON? : Inport  Port=3  LatchInput=off
  Enable : EnablePort  StatesWhenEnabling=reset
  1/mcp : Gain  Gain=1/(mc_mass*mc_cp)  Multiplication=Element-wise(K.*u)  SaturateOnIntegerOverflow=on
  >=0 : Saturate  UpperLimit=Inf  LowerLimit=0  LinearizeAsGain=on
  ">=0 " : Saturate  UpperLimit=Inf  LowerLimit=0  LinearizeAsGain=on
  Block NOTES : Subsystem
      settings: RTWFcnNameOpts=Auto  RTWFileNameOpts=Auto
      mask Display: disp('Block\nNOTES')
  Mux10 : Mux  Inputs=2
      settings: DisplayOption=none
  Mux9 : Mux  Inputs=2
      settings: DisplayOption=none
  Qa : Fcn  Expr=u(1)*(mc_sarea*mc_trq_scale*mc_spd_scale)*u(2)
  Qc1 : Sum  Inputs=-+  SaturateOnIntegerOverflow=on
  Qnet : Sum  Inputs=+++  SaturateOnIntegerOverflow=on
  Qp2a,v7 : Fcn  Expr=amb_tmp-u(1)
  Qr : Fcn  Expr=0.9*(5.67e-8)*(mc_sarea*mc_trq_scale*mc_spd_scale)*((amb_tmp+273)^4 - (u(1)+273)^4)
  Tmc3 : Integrator  ExternalReset=none  InitialConditionSource=internal  InitialCondition=mc_init_tmp  LimitOutput=off  UpperSaturationLimit=inf  LowerSaturationLimit=-inf  ShowSaturationPort=off  ShowStatePort=off  AbsoluteTolerance=auto
  Va/Vv : Gain  Gain=0.5  Multiplication=Element-wise(K.*u)  SaturateOnIntegerOverflow=on
  ha : Fcn  Expr=6 + 6*((abs(u(2))/1000))^0.25 + 60*(abs(u(1))/30)^0.63
  mc coolant : Subsystem  TreatAsAtomicUnit=on
      settings: RTWFcnNameOpts=Auto  RTWFileNameOpts=Auto
  Tmc : Outport  Port=1  InitialOutput=0
  Qmc_clt : Outport  Port=2  OutputWhenDisabled=reset  InitialOutput=0
  wires:
  Mux10/1 -> Qa/1
  Mux9/1 -> ha/1
  Va/Vv/1 -> Mux9/1
  ha/1 -> Mux10/1
  Qp2a,v7/1 -> Mux9/2, Mux10/2
  Qr/1 -> Qnet/3
  Qmc_gen/1 -> ">=0 "/1
  ">=0 "/1 -> Qnet/1
  Qa/1 -> Qnet/2
  veh spd/1 -> Va/Vv/1
  key ON?/1 -> mc coolant/Enable
  >=0/1 -> Qmc_clt/1
  mc coolant/1(Qmc_clt) -> >=0/1, Qc1/1
  Tmc3/1 -> mc coolant/1(Tcl), Tmc/1, Qr/1, Qp2a,v7/1
  1/mcp/1 -> Tmc3/1
  Qc1/1 -> 1/mcp/1
  Qnet/1 -> mc coolant/2("Qmc "), Qc1/2

== system lib_electric_machine/motor/ controller <mc> par/motor controller logic interface ==
  w_mc_out_r : Inport  Port=1  LatchInput=off
  P_mc_in_1lim : Inport  Port=2  LatchInput=off
  P_mc_in_r : Outport  Port=1  InitialOutput=0
  tag scope: P_mc_in_1lim=global, w_mc_out_r=global
  wires:
  P_mc_in_1lim/1 -> [P_mc_in_1lim]
  w_mc_out_r/1 -> [w_mc_out_r]
  [P_mc_in_r] -> P_mc_in_r/1

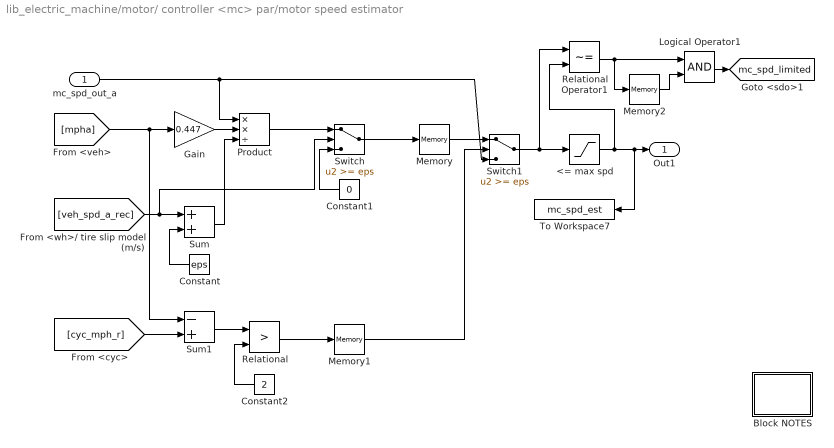
== system lib_electric_machine/motor/ controller <mc> par/motor speed estimator ==
  mc_spd_out_a : Inport  Port=1  LatchInput=off
  <= max spd : Saturate  UpperLimit=max(mc_map_spd)*mc_spd_scale  LowerLimit=-inf  LinearizeAsGain=on
  Block NOTES : Subsystem
      settings: RTWFcnNameOpts=Auto  RTWFileNameOpts=Auto
      mask Display: disp('Block\nNOTES')
  Constant : Constant  Orientation=left  Value=eps
  Constant1 : Constant  Orientation=left  Value=0
  Constant2 : Constant  Orientation=left  Value=2
  Gain : Gain  Gain=0.447  Multiplication=Element-wise(K.*u)  SaturateOnIntegerOverflow=on
  Logical Operator1 : Logic  Operator=AND  Inputs=2
  Memory : Memory  X0=cyc_mph(1,2)*0.447/wh_radius*fd_ratio*max(gb_ratio)*tc_mc_to_fc_ratio  InheritSampleTime=off
      settings: RTWStateStorageClass=Auto
  Memory1 : Memory  X0=1  InheritSampleTime=off
      settings: RTWStateStorageClass=Auto
  Memory2 : Memory  X0=0  InheritSampleTime=off
      settings: RTWStateStorageClass=Auto
  Product : Product  Inputs=**/  Multiplication=Element-wise(.*)  SaturateOnIntegerOverflow=on
  Relational : RelationalOperator  Operator=>
  Relational Operator1 : RelationalOperator  Operator=~=
  Sum : Sum  Inputs=++  SaturateOnIntegerOverflow=on
  Sum1 : Sum  Inputs=-+  SaturateOnIntegerOverflow=on
  Switch : Switch  Threshold=eps
  Switch1 : Switch  Threshold=eps
  To Workspace7 : ToWorkspace  VariableName=mc_spd_est  SampleTime=-1  SaveFormat=Array
  Out1 : Outport  Port=1
  tag scope: mc_spd_limited=global
  wires:
  <= max spd/1 -> Relational Operator1/2, To Workspace7/1, Out1/1
  Switch1/1 -> Relational Operator1/1, <= max spd/1
  Relational Operator1/1 -> Memory2/1, Logical Operator1/1
  Logical Operator1/1 -> [mc_spd_limited]
  Memory2/1 -> Logical Operator1/2
  mc_spd_out_a/1 -> Switch1/3, Product/1
  Product/1 -> Switch/1
  Sum/1 -> Product/3
  Gain/1 -> Product/2
  [veh_spd_a_rec] -> Sum/1, Switch/2
  Constant1/1 -> Switch/3
  Memory/1 -> Switch1/1
  Constant/1 -> Sum/2
  [cyc_mph_r] -> Sum1/2
  [mpha] -> Gain/1, Sum1/1
  Constant2/1 -> Relational/2
  Sum1/1 -> Relational/1
  Relational/1 -> Memory1/1
  Memory1/1 -> Switch1/2
  Switch/1 -> Memory/1

== system lib_electric_machine/motor/ controller <mc> par/rotor drive torque available (Nm) ==
  torque per unit input power (N-m/W) : Inport  Port=1  LatchInput=off
  available input power (W) : Inport  Port=2  LatchInput=off
  Block NOTES : Subsystem
      settings: RTWFcnNameOpts=Auto  RTWFileNameOpts=Auto
      mask Display: disp('Block\nNOTES')
  Constant2 : Constant  Value=inf
  Constant3 : Constant  Value=0
  Product : Product  Inputs=2  Multiplication=Element-wise(.*)  SaturateOnIntegerOverflow=on
  Relational Operator : RelationalOperator  Operator=~=
  Switch : Switch  Threshold=eps
  rotor drive torque available : Outport  Port=1  InitialOutput=0
  wires:
  Constant3/1 -> Switch/3
  Constant2/1 -> Relational Operator/2
  available input power (W)/1 -> Product/2
  Product/1 -> Switch/1
  Relational Operator/1 -> Switch/2
  Switch/1 -> rotor drive torque available/1
  torque per unit input power (N-m/W)/1 -> Product/1, Relational Operator/1

== system lib_electric_machine/motor/ controller <mc> prius/Block NOTES ==
  note: This motor/controller model includes loss data, rotational inertia, and performance limits.
  note: Available torque is computed from available power by assuming that the ratio of rotor torque to input
      | (electric) power is the same for the actual/achievable situation as was computed for the request.  This
      | is mathematically equivalent to assuming that the motor/controller efficiency.  Rotor speed for the
      | actual/achievable calculations is as computed in the 'request' branch.
